simulink library "UI_controller"  (R2020b)
settings: Solver=VariableStepAuto  StartTime=0.0  StopTime=10.0  RelTol=1e-3
settings Model: Creator=priyaD  LastModifiedBy=priyaD

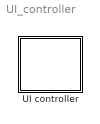
== system UI_controller ==
  UI controller : Stateflow chart  TreatAsAtomicUnit=on

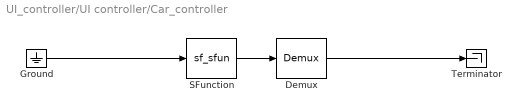
== system UI_controller/UI controller/Car_controller ==
  " Demux " : Demux  Outputs=1
  " Ground " : Ground
  " SFunction " : S-Function  Tag=Stateflow S-Function 1  FunctionName=sf_sfun  PortCounts=[1 1]  SFunctionDeploymentMode=off  EnableBusSupport=off
  " Terminator " : Terminator
  wires:
  " Ground "/1 -> " SFunction "/1
  " Demux "/1 -> " Terminator "/1
  " SFunction "/1 -> " Demux "/1

== stateflow chart UI_controller/UI controller ==
  state Car_controller

== stateflow chart UI_controller/UI controller/Car_controller ==
  state Car_controller
    state close_door [function]
      (default) -> (junction 30) : {ml.sf_lift_gui('close_door',carID);}
    state open_door [function]
      (default) -> (junction 33) : {ml.sf_lift_gui('open_door',carID);}
    state move(pos) [function]
      (default) -> (junction 37) : {ml.sf_lift_gui('move_car',carID,pos);}
    state deactivate_hall_button(pos) [function]
      (default) -> (junction 41) : {ml.sf_lift_gui('deactivate','hall',get_floor_number(pos));}
    state deactivate_car_button(pos) [function]
      (default) -> (junction 45) : {floor_Num=get_floor_number(pos);
          | ml.sf_lif_gui('deactivate',carID,floorNum);}
    state floorNumber = get_floor_number(pos) [function]
      (default) -> (junction 50) : {floorNumber = ml.round(pos);}
    Car_controller -> (junction 2)
    (junction 2) -> (junction 3) [order 1] : [hasChanged(inputPos)]
    (junction 2) -> (junction 4) [order 2]
    (junction 3) -> (junction 5) : {move(inputPos);}
    (junction 5) -> (junction 4)
    (junction 4) -> (junction 6)
    (junction 6) -> (junction 7) [order 1] : [hasChanged(doorOpen)]
    (junction 6) -> (junction 10) [order 2]
    (junction 7) -> (junction 8)
    (junction 8) -> (junction 9) [order 1] : [doorOpen]
    (junction 8) -> (junction 11) [order 2] : {close_door();}
    (junction 9) -> (junction 12) : {open_door();}
    (junction 11) -> (junction 10) : {deactivate_hall_button(inputPos);
        | deactivate_car_button(inpitPos);}
    (junction 12) -> (junction 11)
    (junction 10) -> (junction 13)
  data: pos function_input; pos function_input; pos function_input; pos function_input; floorNumber function_output
